simulink model "battery_linear"  (R2024a)
settings: Solver=VariableStepAuto  StartTime=0.0  StopTime=100000/2  RelTol=1e-3
PreLoadFcn:
  | params_battery;
InitFcn:
  | params_battery;
  | 
  | load('lin_battery.mat','lin');
values from neighbouring files (symbols this model uses):
  lin =     [lin_battery.mat]    (also in linearize_battery_fd.m = struct(); matlab.mat)
  Ts = 0.1    [EKF.m]    (also in params_battery.m)
settings Model: Creator=belit  LastModifiedBy=belit

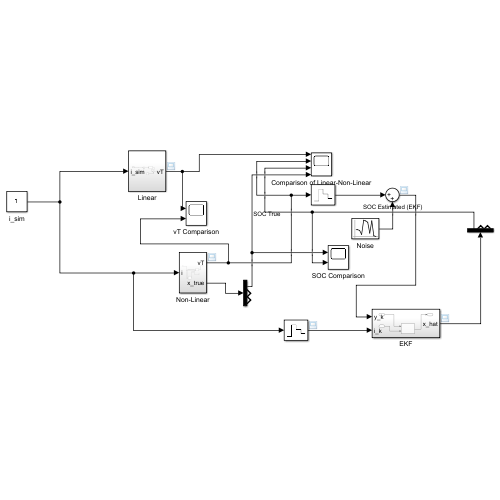
[thumbnail: Simulink's stored preview of the top-level diagram]
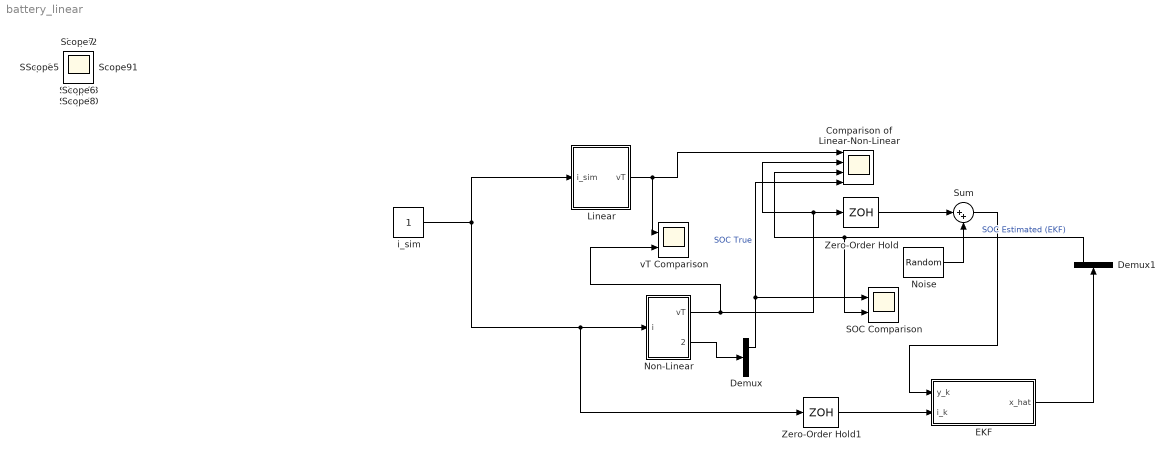
== system battery_linear ==
  Comparison of Linear-Non-Linear : Scope  NumInputPorts=4
  Demux : Demux  Outputs=3
  Demux1 : Demux  Outputs=3
  EKF : Subsystem
  Linear : Subsystem
  Noise : RandomNumber  Variance=1e-4  SampleTime=Ts
  Non-Linear : Subsystem
  SOC Comparison : Scope  NumInputPorts=2
  Sum : Sum  Inputs=|++
  Zero-Order Hold : ZeroOrderHold  SampleTime=Ts
  Zero-Order Hold1 : ZeroOrderHold  SampleTime=Ts
  i_sim : Constant
  vT Comparison : Scope  NumInputPorts=2
  Scope{,1..13} (14 alike) : Scope
  wires:
  i_sim/1 -> Linear/1(i_sim), Zero-Order Hold1/1, Non-Linear/1(i)
  Linear/1(vT) -> vT Comparison/1, Comparison of Linear-Non-Linear/1
  Non-Linear/1(vT) -> vT Comparison/2, Comparison of Linear-Non-Linear/2, Zero-Order Hold/1
  Noise/1 -> Sum/2
  Zero-Order Hold/1 -> Sum/1
  Zero-Order Hold1/1 -> EKF/2(i_k)
  Sum/1 -> EKF/1(y_k)
  Non-Linear/2(x_true) -> Demux/1
  Demux/1 -> SOC Comparison/1, Comparison of Linear-Non-Linear/4  "SOC True"
  EKF/1(x_hat) -> Demux1/1
  Demux1/1 -> SOC Comparison/2, Comparison of Linear-Non-Linear/3  "SOC Estimated (EKF)"

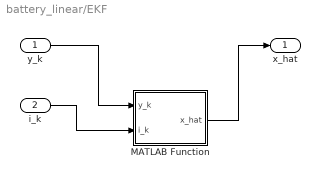
== system battery_linear/EKF ==
  y_k : Inport
  i_k : Inport  Port=2
  MATLAB Function : MATLAB Function  TreatAsAtomicUnit=on
  x_hat : Outport
  wires:
  i_k/1 -> MATLAB Function/2(i_k)
  y_k/1 -> MATLAB Function/1(y_k)
  MATLAB Function/1(x_hat) -> x_hat/1

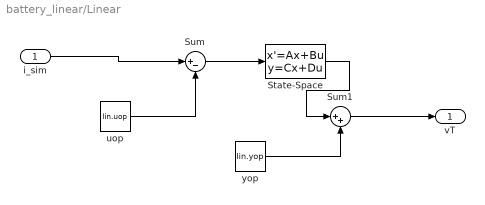
== system battery_linear/Linear ==
  i_sim : Inport
  State-Space : StateSpace  A=lin.A  B=lin.B  C=lin.C  D=lin.D  InitialCondition=[0 0 0]
  Sum : Sum  Inputs=|+-
  Sum1 : Sum  Inputs=|++
  uop : Constant  Value=lin.uop  VectorParams1D=off
  yop : Constant  Value=lin.yop
  vT : Outport
  wires:
  uop/1 -> Sum/2
  yop/1 -> Sum1/2
  State-Space/1 -> Sum1/1
  i_sim/1 -> Sum/1
  Sum/1 -> State-Space/1
  Sum1/1 -> vT/1

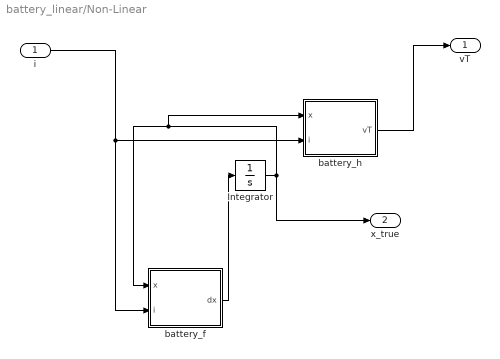
== system battery_linear/Non-Linear ==
  i : Inport
  Integrator : Integrator  InitialCondition=[0.4; 0; 0]
  battery_f : MATLAB Function  TreatAsAtomicUnit=on
  battery_h : MATLAB Function  TreatAsAtomicUnit=on
  vT : Outport
  x_true : Outport  Port=2
  wires:
  i/1 -> battery_f/2(i), battery_h/2(i)
  battery_h/1(vT) -> vT/1
  Integrator/1 -> battery_h/1(x), battery_f/1(x), x_true/1
  battery_f/1(dx) -> Integrator/1

== matlab function battery_linear/Non-Linear/battery_h ==
  data: x input; vT output; i input; theta parameter double size=[25 1]
function vT = fcn(x,i, theta)
vT = battery_h(x,i,theta);
end

== matlab function battery_linear/Non-Linear/battery_f ==
  data: x input; dx output; i input; theta parameter double size=[25 1]
function dx = fcn(x,i, theta)
dx = battery_f(x,i,theta);
end

== matlab function battery_linear/EKF/MATLAB Function ==
  data: y_k input size=[1 1]; x_hat output size=[3 1]; i_k input size=[1 1]; theta parameter
function x_hat = fcn(y_k, i_k, theta)
% EKF for battery model
% States: x = [sigma; vTS; vTL]
% Input:  i_k (A)  discharge is positive
% Meas:   y_k (V)  terminal voltage (noisy)

% --------- tuning / settings ----------
Ts = 0.1;              % sample time (must match your ZOH)
R  = 1e-4;             % measurement variance (10 mV std -> 0.01^2)
Q = diag([1e-9, 1e-6, 1e-6]);   % process noise (higher, trusting) because small noise

% --------- filter memory --------------
persistent x P
if isempty(x)
    x = [0.4; 0; 0];                 % initial estimate (SOC=0.4)
    P = diag([1e-4, 1e-3, 1e-3]);     % initial covariance
end

% --------- PREDICT --------------------
f  = battery_f(x, i_k, theta);        % dx/dt at current estimate
x_pred = x + Ts * f;                  % Euler discretization
x_pred(1) = clamp01(x_pred(1));       % keep SOC in [0,1]

A  = jac_f_fd(x, i_k);                % A = df/dx (3x3)
F  = eye(3) + Ts * A;                 % discrete transition Jacobian
P_pred = F * P * F' + Q;

% Predicted measurement
y_pred = battery_h(x_pred, i_k, theta);

C = jac_h_fd(x_pred, i_k);            % C = dh/dx (1x3)

% --------- UPDATE ---------------------
S = C * P_pred * C' + R;              % innovation covariance (scalar)
K = (P_pred * C') / S;                % Kalman gain (3x1)

x = x_pred + K * (y_k - y_pred);
x(1) = clamp01(x(1));

P = (eye(3) - K * C) * P_pred;

x_hat = x;

% ======================================
% Nested helpers (can see 'theta')
% ======================================

function z = clamp01(z)
    if z < 0
        z = 0;
    elseif z > 1
        z = 1;
    end
end

function A = jac_f_fd(x0, i0)
    % Finite-difference Jacobian of f wrt x
    epsx = 1e-6;
    A = zeros(3,3);
    f0 = battery_f(x0, i0, theta);
    for kk = 1:3
        x1 = x0;
        x1(kk) = x1(kk) + epsx;
        f1 = battery_f(x1, i0, theta);
        A(:,kk) = (f1 - f0) / epsx;
    end
end

function C = jac_h_fd(x0, i0)
    % Finite-difference Jacobian of h wrt x
    epsx = 1e-6;
    C = zeros(1,3);
    y0 = battery_h(x0, i0, theta);
    for kk = 1:3
        x1 = x0;
        x1(kk) = x1(kk) + epsx;
        y1 = battery_h(x1, i0, theta);
        C(1,kk) = (y1 - y0) / epsx;
    end
end

end
